simulink model "simulation_model"  (R2021b)
settings: Solver=VariableStepAuto  StartTime=0.0  StopTime=10.0  RelTol=1e-3
values from neighbouring files (symbols this model uses):
  x0 = [0 0 deg2rad(0) -slider.xwidth/2 -0.02]'    [nonlinear_model_simulation.m]
settings Model: Creator=workstation  LastModifiedBy=Marco
settings SolverCC: AlgebraicLoopSolver=TrustRegion
settings DataIOCC: ReturnWorkspaceOutputs=off
settings DebuggingCC: SFMachineParentedDataDiag=warning  ArithmeticOperatorsInVariantConditions=warning
settings SFSimCC: CustomCodeUndefinedFunction=UseInterfaceOnly

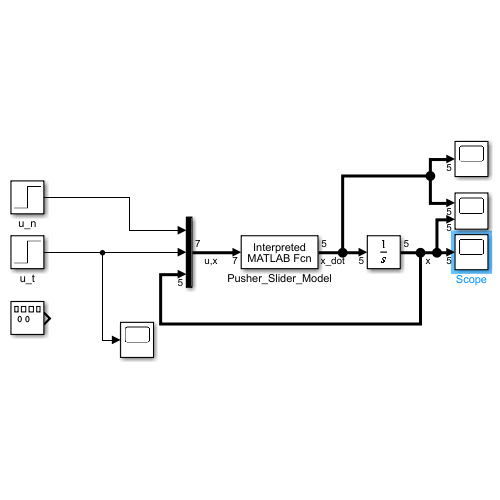
[thumbnail: Simulink's stored preview of the top-level diagram]
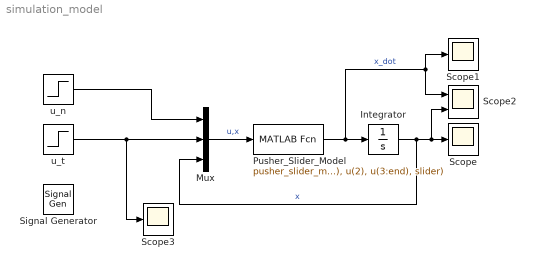
== system simulation_model ==
  Integrator : Integrator  InitialCondition=x0
  Mux : Mux  Inputs=[1 1 5]
  Pusher_Slider_Model : MATLABFcn  MATLABFcn=pusher_slider_model(u(1), u(2), u(3:end), slider)  OutputDimensions=5
  Scope : Scope
  Scope1 : Scope
  Scope2 : Scope  NumInputPorts=2
  Scope3 : Scope
  Signal Generator : SignalGenerator  Amplitude=0.03  Units=rad/sec
  u_n : Step  Before=0.032  After=0.032  SampleTime=0
  u_t : Step  After=0  SampleTime=0
  wires:
  Mux/1 -> Pusher_Slider_Model/1  "u,x"
  Pusher_Slider_Model/1 -> Scope2/1, Scope1/1, Integrator/1  "x_dot"
  Integrator/1 -> Scope2/2, Scope/1, Mux/3  "x"
  u_n/1 -> Mux/1
  u_t/1 -> Scope3/1, Mux/2
